simulink model "Led_Blink"  (R2013a)
settings: Solver=FixedStepDiscrete  StartTime=0.0  StopTime=inf  FixedStep=0.01  RelTol=1e-3
settings Model: Creator=IJ1  LastModifiedBy=IJ1
settings HardwareCC: ProdLargestAtomicInteger=Long  ProdLargestAtomicFloat=Double  ProdEndianess=LittleEndian  ProdHWDeviceType=ARM Compatible->ARM Cortex
settings RTWCC: GenerateReport=on  CustomHeaderCode=#include <wiringPi.h>  LaunchReport=on
settings RTWCC: CustomInitializer=|
  | pinMode (0, OUTPUT) ;
  |  pinMode (1, INPUT) ;
  |  pullUpDnControl(1, PUD_UP);

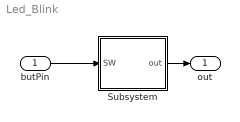
== system Led_Blink ==
  butPin : Inport
  Subsystem : Subsystem  TreatAsAtomicUnit=on
  out : Outport
  wires:
  butPin/1 -> Subsystem/1(SW)
  Subsystem/1(out) -> out/1

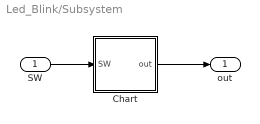
== system Led_Blink/Subsystem ==
  SW : Inport
  Chart : Stateflow chart  TreatAsAtomicUnit=on
  out : Outport
  wires:
  Chart/1(out) -> out/1
  SW/1 -> Chart/1(SW)

== stateflow chart Led_Blink/Subsystem/Chart ==
  state OFF
    en: out=0;
    printf("LED_OFF\r\n");
  state ON
    en: out =1;
    printf("LED_ON\r\n");
  (default) -> ON
  OFF -> ON : [SW==1]
      | /*LED_on*/
  ON -> OFF : [SW==0]
      | /*LED_off*/
  data: SW input; out output double
